simulink model "LMI"  (R2025b)
settings: Solver=VariableStepAuto  StartTime=0.0  StopTime=20.0  RelTol=1e-3
undefined symbols (not defined in the file): A, B, K_LMI, N, X0, x_ref
settings Model: Creator=salvo  LastModifiedBy=salvo

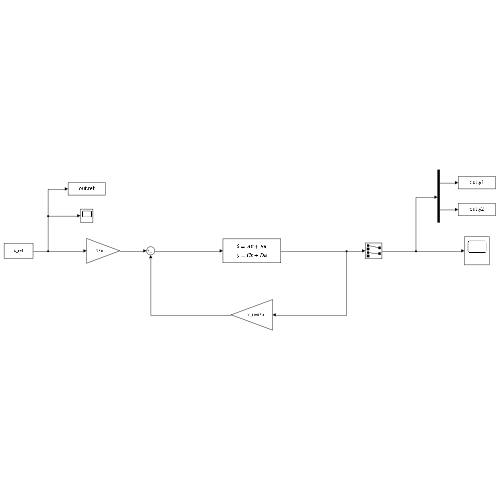
[thumbnail: Simulink's stored preview of the top-level diagram]
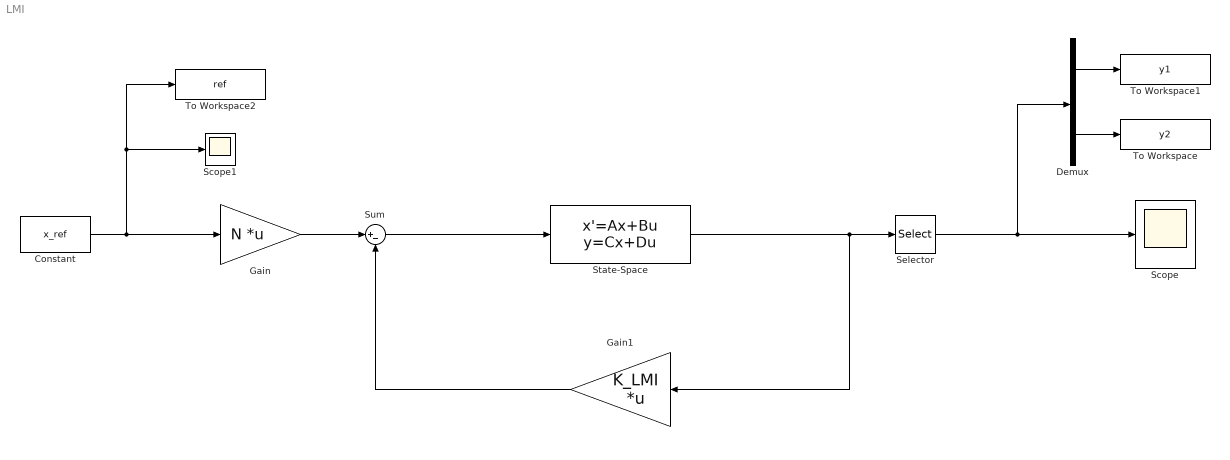
== system LMI ==
  Constant : Constant  Value=x_ref
  Demux : Demux  Outputs=2
  Gain : Gain  Gain=N  Multiplication=Matrix(K*u)
  Gain1 : Gain  Gain=K_LMI  Multiplication=Matrix(K*u)
  Scope : Scope
      settings: ActiveDisplayYMinimum=0.015676347685689124  ActiveDisplayYMaximum=0.28439975776047377
  Scope1 : Scope
  Selector : Selector  InputPortWidth=4  IndexOptions=Index vector (dialog)  Indices=[1 3]  OutputSizes=1
  State-Space : StateSpace  A=A  B=B  C=eye(4)  D=zeros(4,1)  InitialCondition=X0
  Sum : Sum  Inputs=|+-
  To Workspace : ToWorkspace  VariableName=y2  SaveFormat=Timeseries  SampleTime=-1
  To Workspace1 : ToWorkspace  VariableName=y1  SaveFormat=Timeseries  SampleTime=-1
  To Workspace2 : ToWorkspace  VariableName=ref  SaveFormat=Timeseries  SampleTime=-1
  wires:
  Sum/1 -> State-Space/1
  Gain1/1 -> Sum/2
  Gain/1 -> Sum/1
  State-Space/1 -> Selector/1, Gain1/1
  Selector/1 -> Demux/1, Scope/1
  Demux/1 -> To Workspace1/1
  Demux/2 -> To Workspace/1
  Constant/1 -> Gain/1, Scope1/1, To Workspace2/1
